simulink model "optsim1"  (R2022a)
settings: Solver=ode5  StartTime=0.0  StopTime=100  FixedStep=1  MaxStep=0.1  RelTol=1e-3  AbsTol=1e-6
PreLoadFcn:
  | a1=3; a2=43;
PostLoadFcn:
  | optsiminit
values from neighbouring files (symbols this model uses):
  Kd = global_best_position(3)    [PSO.m]    (also in tracklsq.m = pid(3))
  Kp = global_best_position(1)    [PSO.m]    (also in tracklsq.m = pid(1))
settings Model: ExtModeTrigMode=oneshot  ExtModeArmWhenConnect=off  Creator=nikita  LastModifiedBy=mjsung2
settings SolverCC: AutoScaleAbsTol=off  AlgebraicLoopSolver=TrustRegion
settings DataIOCC: SaveFormat=Array  SignalLoggingSaveFormat=ModelDataLogs  SaveTime=off  ReturnWorkspaceOutputs=off  StateSaveName=x  TimeSaveName=t
settings OptimizationCC: BooleanDataType=off  InitFltsAndDblsToZero=on  LifeSpan=inf
settings DebuggingCC: SaveWithParameterizedLinksMsg=none  UnderspecifiedInitializationDetection=Classic  MergeDetectMultiDrivingBlocksExec=none  SignalResolutionControl=TryResolveAllWithWarning  MultiTaskDSMMsg=warning  MultiTaskCondExecSysMsg=none  IntegerOverflowMsg=none  FcnCallInpInsideContextMsg=warning  UnconnectedInputMsg=warning  UnconnectedOutputMsg=warning  UnconnectedLineMsg=warning  SFUnexpectedBacktrackingDiag=warning  SFNoUnconditionalDefaultTransitionDiag=warning  SFExecutionAtInitializationDiag=none  SFMachineParentedDataDiag=warning  IntegerSaturationMsg=none  ArithmeticOperatorsInVariantConditions=warning
settings HardwareCC: ProdBitPerPointer=32  ProdBitPerSizeT=32  ProdBitPerPtrDiffT=32  ProdLargestAtomicFloat=None  ProdIntDivRoundTo=Undefined  ProdEndianess=Unspecified  ProdWordSize=32  ProdHWDeviceType=32-bit Generic  TargetUnknown=on
settings ModelReferenceCC: PropagateSignalLabelsOutOfModel=off
settings SFSimCC: SimUseLocalCustomCode=off  CustomCodeUndefinedFunction=UseInterfaceOnly
settings RTWCC: RTWUseLocalCustomCode=off
settings CodeAppCC: StateflowObjectComments=on
settings GRTTargetCC: TargetFcnLib=ansi_tfl_tmw.mat  TargetLangStandard=C89/C90 (ANSI)  CombineOutputUpdateFcns=off  GRTInterface=on
settings ConfigComp: CovMetricSettings=dw  CovSaveCumulativeToWorkspaceVar=on  CovSaveSingleToWorkspaceVar=on  CovExternalEMLEnable=off

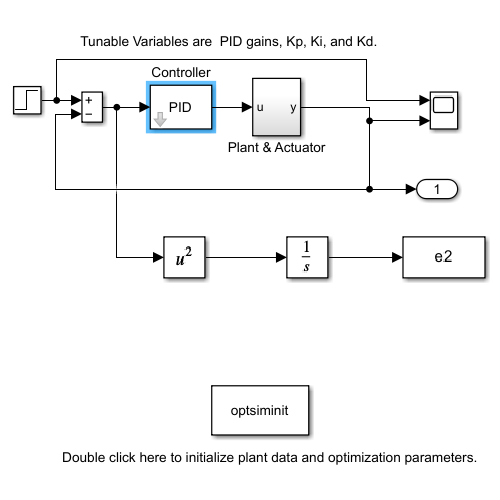
[thumbnail: Simulink's stored preview of the top-level diagram]
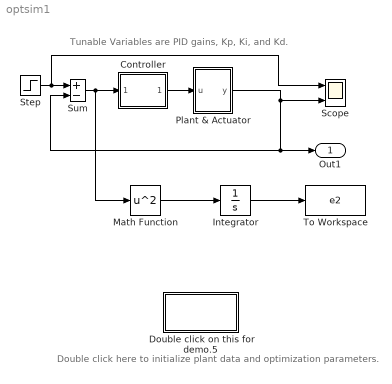
== system optsim1 ==
  note: Double click here to initialize plant data and optimization parameters.
  note: Tunable Variables are PID gains, Kp, Ki, and Kd.
  Controller : Subsystem  mask(PID Controller){P=Kp, I=0, D=Kd}
      mask prompts: P "Proportional:"; I "Integral"; D "Derivative:"
      mask help: Enter expressions for proportional, integral, and derivative terms.
      mask Help: This block implements a PID controller where paramaters are entered for the Proportional, Integral and Derivative terms.
      mask Display: disp('PID')
  Double click on this for demo.5 : Subsystem
      settings: OpenFcn=optsiminit
      mask Display: disp('optsiminit')
  Integrator : Integrator
  Math Function : Math  Operator=square  SignedPower=on
  Plant & Actuator : Subsystem
  Scope : Scope  NumInputPorts=2
  Step : Step  Time=0  SampleTime=0
  Sum : Sum  Inputs=+-  InputSameDT=on  SaturateOnIntegerOverflow=on  OutDataTypeStr=Inherit: Same as first input
  To Workspace : ToWorkspace  VariableName=e2  SampleTime=-1
      settings: MaxDataPoints=1
  Out1 : Outport  VectorParamsAs1DForOutWhenUnconnected=off
  wires:
  Plant & Actuator/1(y) -> Sum/2, Out1/1, Scope/2
  Sum/1 -> Controller/1(In_1), Math Function/1
  Step/1 -> Scope/1, Sum/1
  Controller/1(Out_1) -> Plant & Actuator/1("u ")
  Math Function/1 -> Integrator/1
  Integrator/1 -> To Workspace/1

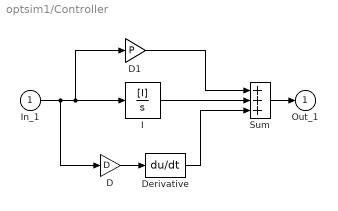
== system optsim1/Controller ==
  In_1 : Inport
  D : Gain  Gain=D  SaturateOnIntegerOverflow=on  OutDataTypeStr=Inherit: Same as input  ParamDataTypeStr=Inherit: Same as input
  D1 : Gain  Gain=P  SaturateOnIntegerOverflow=on  OutDataTypeStr=Inherit: Same as input  ParamDataTypeStr=Inherit: Same as input
  Derivative : Derivative
  I : TransferFcn  Numerator=[I]  Denominator=[1 0]
  Sum : Sum  Inputs=+++  InputSameDT=on  SaturateOnIntegerOverflow=on  OutDataTypeStr=Inherit: Same as first input
  Out_1 : Outport  InitialOutput=0  VectorParamsAs1DForOutWhenUnconnected=off
  wires:
  In_1/1 -> D1/1, I/1, D/1
  Sum/1 -> Out_1/1
  D/1 -> Derivative/1
  Derivative/1 -> Sum/3
  I/1 -> Sum/2
  D1/1 -> Sum/1

== system optsim1/Double click on this for demo.5 ==

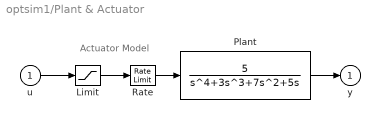
== system optsim1/Plant & Actuator ==
  note: Actuator Model
  "u " : Inport
  Limit : Saturate  UpperLimit=2  LowerLimit=-2
  Plant : TransferFcn  Numerator=[5]  Denominator=[1 3 7 5 0]
  Rate : RateLimiter  RisingSlewLimit=0.8  FallingSlewLimit=-0.8
  y : Outport  InitialOutput=0  VectorParamsAs1DForOutWhenUnconnected=off
  wires:
  Plant/1 -> y/1
  "u "/1 -> Limit/1
  Rate/1 -> Plant/1
  Limit/1 -> Rate/1
